simulink model "chap4_1sim"  (Simulink 7.7)
settings: Solver=ode45  StartTime=0.0  StopTime=3  FixedStep=0.001  RelTol=1e-3
settings Model: Creator=ljk  LastModifiedBy=ljk  ExtModeTrigMode=oneshot  ExtModeArmWhenConnect=off
settings DataIOCC: LimitDataPoints=off  SignalLoggingName=sigsOut
settings OptimizationCC: BooleanDataType=off
settings DebuggingCC: SaveWithParameterizedLinksMsg=none  SignalResolutionControl=TryResolveAllWithWarning  SolverPrmCheckMsg=none  MultiTaskDSMMsg=warning  MultiTaskCondExecSysMsg=none  StrictBusMsg=None
settings HardwareCC: TargetUnknown=on
settings RTWCC: IncludeERTFirstTime=on

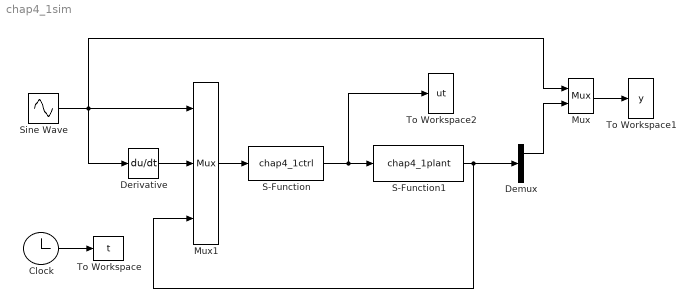
== system chap4_1sim ==
  Clock : Clock
  Demux : Demux  Outputs=3
  Derivative : Derivative
  Mux : Mux  Inputs=2
  Mux1 : Mux  Inputs=3
  S-Function : S-Function  FunctionName=chap4_1ctrl  EnableBusSupport=off
  S-Function1 : S-Function  FunctionName=chap4_1plant  EnableBusSupport=off
  Sine Wave : Sin  Amplitude=5  Frequency=2*pi  SampleTime=0
  To Workspace : ToWorkspace  VariableName=t  SampleTime=-1  SaveFormat=Array
  To Workspace1 : ToWorkspace  VariableName=y  SampleTime=-1  SaveFormat=Array
  To Workspace2 : ToWorkspace  VariableName=ut  SampleTime=-1  SaveFormat=Array
  wires:
  Mux1/1 -> S-Function/1
  S-Function/1 -> S-Function1/1, To Workspace2/1
  Derivative/1 -> Mux1/2
  Sine Wave/1 -> Mux/1, Mux1/1, Derivative/1
  Mux/1 -> To Workspace1/1
  Demux/1 -> Mux/2
  S-Function1/1 -> Demux/1, Mux1/3
  Clock/1 -> To Workspace/1
